simulink model "CellElement"  (R2012b)
settings: Solver=ode45  StartTime=0.0  StopTime=10.0  RelTol=1e-3
settings Model: Creator=sz609516  LastModifiedBy=sz609516
settings DataIOCC: SignalLoggingSaveFormat=ModelDataLogs
settings DebuggingCC: FcnCallInpInsideContextMsg=EnableAllAsWarning
settings GRTTargetCC: CombineOutputUpdateFcns=off  GRTInterface=on

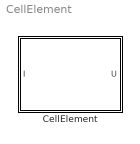
== system CellElement ==
  CellElement : Subsystem

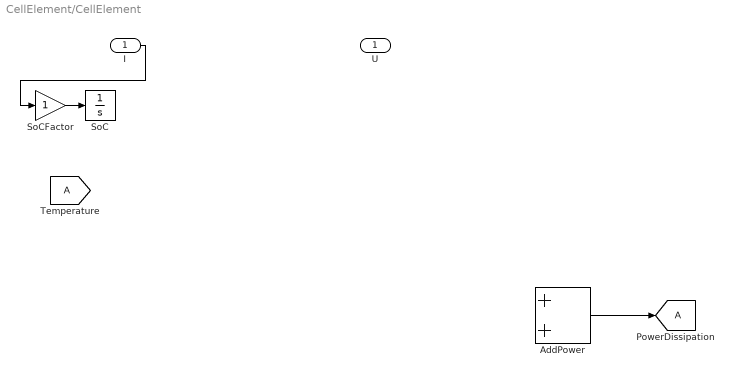
== system CellElement/CellElement ==
  I : Inport
  AddPower : Sum
  SoC : Integrator
  SoCFactor : Gain
  U : Outport
  tag scope: A=global
  wires:
  AddPower/1 -> [A]
  I/1 -> SoCFactor/1
  SoCFactor/1 -> SoC/1
